simulink model "position_control_dc"  (R2022b)
settings: Solver=VariableStepAuto  StartTime=0.0  StopTime=10.0  RelTol=1e-3
undefined symbols (not defined in the file): a, b, Kd, Kp
settings Model: Creator=sokse  LastModifiedBy=sokse

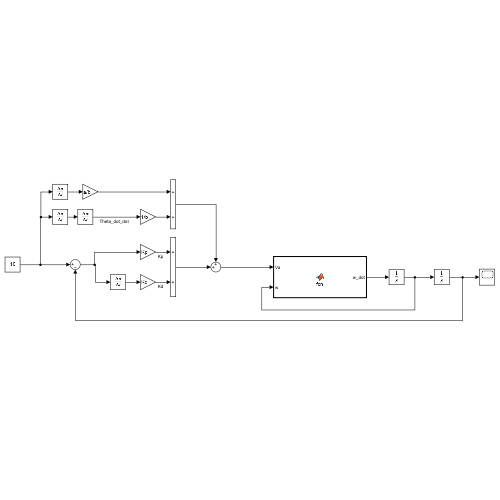
[thumbnail: Simulink's stored preview of the top-level diagram]
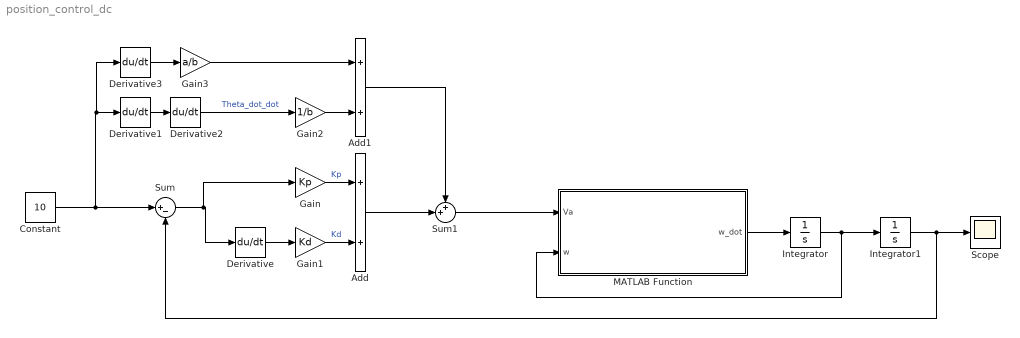
== system position_control_dc ==
  Add : Sum
  Add1 : Sum
  Constant : Constant  Value=10
  Derivative{,1..3} (4 alike) : Derivative
  Gain : Gain  Gain=Kp
  Gain1 : Gain  Gain=Kd
  Gain2 : Gain  Gain=1/b
  Gain3 : Gain  Gain=a/b
  Integrator : Integrator
  Integrator1 : Integrator
  MATLAB Function : MATLAB Function  TreatAsAtomicUnit=on
  Scope : Scope
  Sum : Sum  Inputs=|+-
  Sum1 : Sum  Inputs=++|
  wires:
  MATLAB Function/1(w_dot) -> Integrator/1
  Integrator/1 -> MATLAB Function/2(w), Integrator1/1
  Integrator1/1 -> Sum/2, Scope/1
  Constant/1 -> Derivative3/1, Derivative1/1, Sum/1
  Derivative/1 -> Gain1/1
  Sum/1 -> Gain/1, Derivative/1
  Gain/1 -> Add/1  "Kp"
  Gain1/1 -> Add/2  "Kd"
  Add/1 -> Sum1/2
  Sum1/1 -> MATLAB Function/1(Va)
  Derivative1/1 -> Derivative2/1
  Derivative2/1 -> Gain2/1  "Theta_dot_dot"
  Derivative3/1 -> Gain3/1
  Gain3/1 -> Add1/1
  Gain2/1 -> Add1/2
  Add1/1 -> Sum1/1

== matlab function position_control_dc/MATLAB Function ==
  data: Va input; w_dot output; w input
function w_dot = fcn(Va,w)

a = 10; 
b = 25; 
w_dot = -a*w+b*Va;
